simulink model "cruise_open_loop_discrete"  (R2024a)
settings: Solver=VariableStepAuto  StartTime=0.0  StopTime=700  RelTol=1e-3
settings Model: Creator=root  LastModifiedBy=kiran m v
settings SolverCC: AlgebraicLoopSolver=TrustRegion
settings DataIOCC: ReturnWorkspaceOutputs=off
settings DebuggingCC: UnconnectedInputMsg=warning  UnconnectedOutputMsg=warning  UnconnectedLineMsg=warning  ArithmeticOperatorsInVariantConditions=warning
settings ModelReferenceCC: EnableRefExpFcnMdlSchedulingChecks=on
settings SFSimCC: SimUseLocalCustomCode=off  CustomCodeUndefinedFunction=UseInterfaceOnly
settings RTWCC: RTWUseLocalCustomCode=off  GPUComputeCapability=3.5
settings CodeAppCC: StateflowObjectComments=on

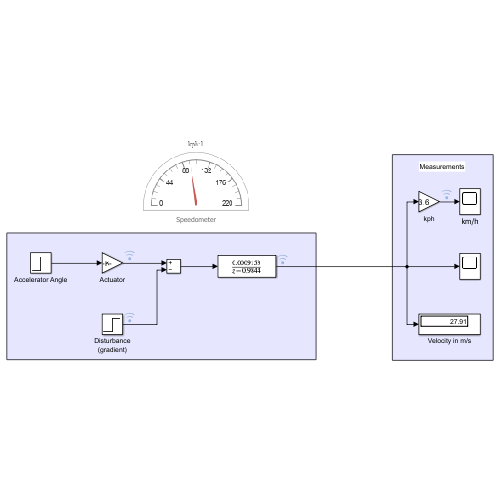
[thumbnail: Simulink's stored preview of the top-level diagram]
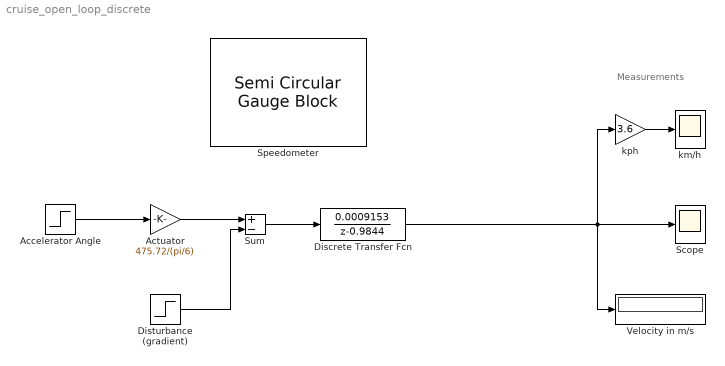
== system cruise_open_loop_discrete ==
  note: Measurements
  Accelerator Angle : Step  After=pi/6  SampleTime=0
  Actuator : Gain  Gain=475.72/(pi/6)
  Discrete Transfer Fcn : DiscreteTransferFcn  Numerator=[0.0009153]  Denominator=[1 -0.9844]  SampleTime=1
  Disturbance (gradient) : Step  Time=800  After=475.72*9.81*sin(pi/45)  SampleTime=0
  Scope : Scope
  Speedometer : SemiCircularGaugeBlock  ScaleMax=220
  Sum : Sum  Inputs=+-
  Velocity in m/s : Display
  km/h : Scope
  kph : Gain  Gain=3.6
  wires:
  Discrete Transfer Fcn/1 -> kph/1, Velocity in m/s/1, Scope/1
  Disturbance (gradient)/1 -> Sum/2
  Actuator/1 -> Sum/1
  Sum/1 -> Discrete Transfer Fcn/1
  Accelerator Angle/1 -> Actuator/1
  kph/1 -> km/h/1
